simulink model "Areodynamic_Coefficient"  (R2022a)
settings: Solver=VariableStepAuto  StartTime=0.0  StopTime=1  RelTol=1e-3
undefined symbols (not defined in the file): a1, ac, AeroCoeff, b1
libraries: aerolibconvert2 x4
(part 2 of 2)

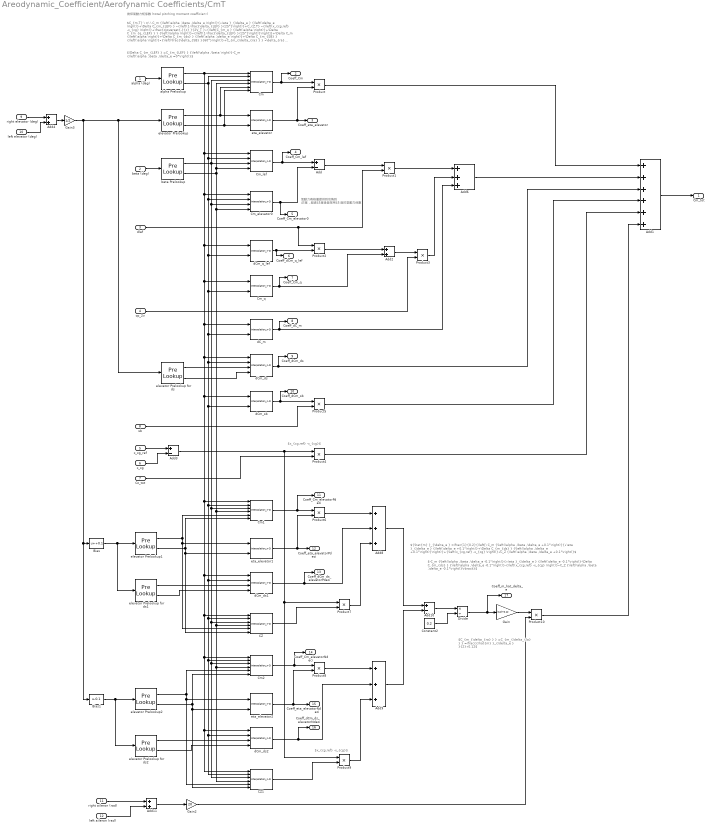
== system Areodynamic_Coefficient/Aerofynamic Coefficients/CmT ==
  note: 氣動力表格僅提供到攻角到
      | 45度，超過45度後皆採用45
      | 度的氣動力係數
  note: $x_{cg,ref} -x_{cg}$
  note: 俯仰氣動力矩係數 (total pitching moment coefficient)：
  note: $\Delta C_{m_{LEF} } =C_{m_{LEF} } {\left(\alpha ,\beta \right)}-C_m {\left(\alpha ,\beta ,\delta_e =0°\right)}$
  note: $C_{m,T} \ =\ \ C_m {\left(\alpha ,\beta ,\delta_e \right)}{∙\eta }_{\delta_e } {\left(\delta_e \right)}+\Delta C_{m_{LEF} } ∙{\left(1-\frac{\delta_{LEF} }{25°}\right)}+C_{Z,T} ∙{\left(x_{cg,ref} -x_{cg} \right)}+\frac{q\overset{-}{c} }{2V_T }∙{\left[C_{m_q } {\left(\alpha \right)}+\Delta C_{m_{q_{LEF} } } {\left(\alpha \right)}∙{\left(1-\frac{\delta_{LEF} }{25°}\right)}\right]}+\Delta C_m {\left(\alpha \right)}+\Delta C_{m_{ds} } {\left(\alpha ,\delta_e \right)}+\Delta C_{m_{SB} } {\left(\alpha \right)}∙{\left(\frac{\delta_{SB} }{60°}\right)}+C_{m_{\delta_{ra} } } ∙\delta_{ra} +C_{m_{\delta_{la} } } ∙\delta_{la}$
  note: $-C_m {\left(\alpha ,\beta ,\delta_e -0.1°\right)}{∙\eta }_{\delta_e } {\left(\delta_e -0.1°\right)}-\Delta C_{m_{ds} } {\left(\alpha ,\delta_e -0.1°\right)}-{\left(x_{cg,ref} -x_{cg} \right)}∙C_Z {\left(\alpha ,\beta ,\delta_e -0.1°\right)}\rbrack}$
  note: ${\hat{m} }_{\delta_e } =\frac{1}{0.2}{\left[\ C_m {\left(\alpha ,\beta ,\delta_e +0.1°\right)}{∙\eta }_{\delta_e } {\left(\delta_e +0.1°\right)}+\Delta C_{m_{ds} } {\left(\alpha ,\delta_e +0.1°\right)}\right)}+{\left(x_{cg,ref} -x_{cg} \right)}∙C_Z {\left(\alpha ,\beta ,\delta_e +0.1°\right)}$
  note: $x_{cg,ref} -x_{cg}$
  note: $C_{m_{\delta_{ra} } } =C_{m_{\delta_{la} } } =\frac{{\hat{m} }_{\delta_e } }{2}∙0.12$
  alpha (deg) : Inport
  beta (deg) : Inport  Port=2
  dlef : Inport  Port=3
  qc_2v : Inport  Port=4
  x_cg_ref : Inport  Port=5
  x_cg : Inport  Port=6
  Cz_tot : Inport  Port=7
  sb : Inport  Port=8
  right elevator (deg) : Inport  Port=9
  left elevator (deg) : Inport  Port=10
  right aileron (rad) : Inport  Port=11
  left aileron (rad) : Inport  Port=12
  Add : Sum  Inputs=+-
  Add1 : Sum  Inputs=++++++
  Add10 : Sum  Inputs=+-
  Add11 : Sum
  Add2 : Sum
  Add3 : Sum  Inputs=+-
  Add4 : Sum
  Add6 : Sum  Inputs=+++
  Add8 : Sum  Inputs=+++
  Add9 : Sum  Inputs=+++
  Bias : Bias  Bias=+0.1  SaturateOnIntegerOverflow=off
  Bias1 : Bias  Bias=-0.1  SaturateOnIntegerOverflow=off
  CZ : Interpolation_n-D  NumberOfTableDimensions=3  Table=AeroCoeff.CZ
      settings: InputPortMap=u0,u1,u2,u3,u4,u5
  CZ1 : Interpolation_n-D  NumberOfTableDimensions=3  Table=AeroCoeff.CZ
      settings: InputPortMap=u0,u1,u2,u3,u4,u5
  Cm : Interpolation_n-D  NumberOfTableDimensions=3  Table=AeroCoeff.Cm
      settings: InputPortMap=u0,u1,u2,u3,u4,u5
  Cm1 : Interpolation_n-D  NumberOfTableDimensions=3  Table=AeroCoeff.Cm
      settings: InputPortMap=u0,u1,u2,u3,u4,u5
  Cm2 : Interpolation_n-D  NumberOfTableDimensions=3  Table=AeroCoeff.Cm
      settings: InputPortMap=u0,u1,u2,u3,u4,u5
  Cm_elevator0 : Interpolation_n-D  Table=AeroCoeff.Cm_elevator0
  Cm_lef : Interpolation_n-D  Table=AeroCoeff.Cm_lef
  Cm_q : Interpolation_n-D  NumberOfTableDimensions=1  Table=AeroCoeff.Cm_q
      settings: InputPortMap=u0,u1
  Constant2 : Constant  Value=0.2
  Divide : Product  Inputs=*/
  Gain : Gain  Gain=(1/2)*0.12
  Gain2 : Gain  Gain=20
  Gain3 : Gain  Gain=1/2
  Product{,1..10} (11 alike) : Product
  alpha Prelookup : PreLookup  BreakpointsData=AeroCoeff.alpha_prelookup  IndexSearchMethod=Linear search  BeginIndexSearchUsingPreviousIndexResult=on  DiagnosticForOutOfRangeInput=Warning
  beta Prelookup : PreLookup  BreakpointsData=AeroCoeff.beta_prelookup  IndexSearchMethod=Linear search  BeginIndexSearchUsingPreviousIndexResult=on  DiagnosticForOutOfRangeInput=Warning
  dC_m : Interpolation_n-D  NumberOfTableDimensions=1  Table=AeroCoeff.dC_m
      settings: InputPortMap=u0,u1
  dCm_ds : Interpolation_n-D  Table=AeroCoeff.dCm_ds
  dCm_ds1 : Interpolation_n-D  Table=AeroCoeff.dCm_ds
  dCm_ds2 : Interpolation_n-D  Table=AeroCoeff.dCm_ds
  dCm_q_lef : Interpolation_n-D  NumberOfTableDimensions=1  Table=AeroCoeff.dCm_q_lef
      settings: InputPortMap=u0,u1
  dCm_sb : Interpolation_n-D  NumberOfTableDimensions=1  Table=AeroCoeff.dCm_sb
      settings: InputPortMap=u0,u1
  elevator Prelookup : PreLookup  BreakpointsData=AeroCoeff.elevator_prelookup2  IndexSearchMethod=Linear search  BeginIndexSearchUsingPreviousIndexResult=on  DiagnosticForOutOfRangeInput=Warning
  elevator Prelookup for ds : PreLookup  BreakpointsData=AeroCoeff.elevator_prelookup3  IndexSearchMethod=Linear search  BeginIndexSearchUsingPreviousIndexResult=on  DiagnosticForOutOfRangeInput=Warning
  elevator Prelookup for ds1 : PreLookup  BreakpointsData=AeroCoeff.elevator_prelookup3  IndexSearchMethod=Linear search  BeginIndexSearchUsingPreviousIndexResult=on  DiagnosticForOutOfRangeInput=Warning
  elevator Prelookup for ds2 : PreLookup  BreakpointsData=AeroCoeff.elevator_prelookup3  IndexSearchMethod=Linear search  BeginIndexSearchUsingPreviousIndexResult=on  DiagnosticForOutOfRangeInput=Warning
  elevator Prelookup1 : PreLookup  BreakpointsData=AeroCoeff.elevator_prelookup2  IndexSearchMethod=Linear search  BeginIndexSearchUsingPreviousIndexResult=on  DiagnosticForOutOfRangeInput=Warning
  elevator Prelookup2 : PreLookup  BreakpointsData=AeroCoeff.elevator_prelookup2  IndexSearchMethod=Linear search  BeginIndexSearchUsingPreviousIndexResult=on  DiagnosticForOutOfRangeInput=Warning
  eta_elevator : Interpolation_n-D  NumberOfTableDimensions=1  Table=AeroCoeff.eta_elevator
      settings: InputPortMap=u0,u1
  eta_elevator1 : Interpolation_n-D  NumberOfTableDimensions=1  Table=AeroCoeff.eta_elevator
      settings: InputPortMap=u0,u1
  eta_elevator2 : Interpolation_n-D  NumberOfTableDimensions=1  Table=AeroCoeff.eta_elevator
      settings: InputPortMap=u0,u1
  Cm_tot : Outport  VectorParamsAs1DForOutWhenUnconnected=off
  Coeff_Cm : Outport  Port=2
  Coeff_eta_elevator : Outport  Port=3
  Coeff_Cm_lef : Outport  Port=4
  Coeff_Cm_elevator0 : Outport  Port=5
  Coeff_dCm_q_lef : Outport  Port=6
  Coeff_Cm_q : Outport  Port=7
  Coeff_dC_m : Outport  Port=8
  Coeff_dCm_ds : Outport  Port=9
  Coeff_dCm_sb : Outport  Port=10
  Coeff_Cm_elevatorPdeci : Outport  Port=11
  Coeff_eta_elevatorPdeci : Outport  Port=12
  Coeff_dCm_ds_elevatorPdeci : Outport  Port=13
  Coeff_Cm_elevatorNdeci : Outport  Port=14
  Coeff_eta_elevatorNdeci : Outport  Port=15
  Coeff_dCm_ds_elevatorNdeci : Outport  Port=16
  Coeff_m_hat_delta_e : Outport  Port=17
  wires:
  Cm_lef/1 -> Coeff_Cm_lef/1, Add/1
  Add3/1 -> Product4/1, Product7/1, Product9/1
  alpha Prelookup/1 -> Cm1/1, dCm_ds2/1, CZ1/1, Cm2/1, CZ/1, dCm_ds1/1, dCm_sb/1, dCm_ds/1, dC_m/1, Cm_q/1, dCm_q_lef/1, Cm_elevator0/1, Cm_lef/1, Cm/1
  Cm_elevator0/1 -> Coeff_Cm_elevator0/1, Add/2
  elevator Prelookup/1 -> eta_elevator/1, Cm/5
  dC_m/1 -> Coeff_dC_m/1, Add6/3
  alpha Prelookup/2 -> Cm1/2, dCm_ds1/2, Cm2/2, dCm_ds2/2, CZ1/2, CZ/2, dCm_sb/2, dCm_ds/2, dC_m/2, Cm_q/2, dCm_q_lef/2, Cm_elevator0/2, Cm_lef/2, Cm/2
  dlef/1 -> Product2/1, Product1/2
  elevator Prelookup/2 -> eta_elevator/2, Cm/6
  Add4/1 -> Gain3/1
  eta_elevator/1 -> Coeff_eta_elevator/1, Product/2
  beta Prelookup/2 -> Cm/4, Cm_lef/4, Cm1/4, CZ/4, Cm2/4, CZ1/4, Cm_elevator0/4
  Product2/1 -> Add2/1
  Cm_q/1 -> Coeff_Cm_q/1, Add2/2
  beta Prelookup/1 -> Cm/3, Cm1/3, CZ/3, Cm2/3, CZ1/3, Cm_elevator0/3, Cm_lef/3
  dCm_q_lef/1 -> Coeff_dCm_q_lef/1, Product2/2
  Add2/1 -> Product3/1
  Add/1 -> Product1/1
  qc_2v/1 -> Product3/2
  alpha (deg)/1 -> alpha Prelookup/1
  Product4/1 -> Add1/5
  beta (deg)/1 -> beta Prelookup/1
  x_cg/1 -> Add3/2
  Add1/1 -> Cm_tot/1
  Cz_tot/1 -> Product4/2
  x_cg_ref/1 -> Add3/1
  sb/1 -> Product5/2
  dCm_sb/1 -> Coeff_dCm_sb/1, Product5/1
  Product5/1 -> Add1/4
  elevator Prelookup for ds/1 -> dCm_ds/3
  elevator Prelookup for ds/2 -> dCm_ds/4
  dCm_ds/1 -> Coeff_dCm_ds/1, Add1/3
  Product1/1 -> Add6/1
  Product3/1 -> Add6/2
  Add6/1 -> Add1/2
  Product/1 -> Add1/1
  right elevator (deg)/1 -> Add4/1
  left elevator (deg)/1 -> Add4/2
  eta_elevator1/1 -> Product6/2, Coeff_eta_elevatorPdeci/1
  Cm1/1 -> Coeff_Cm_elevatorPdeci/1, Product6/1
  elevator Prelookup1/1 -> Cm1/5, eta_elevator1/1, CZ/5
  elevator Prelookup1/2 -> Cm1/6, eta_elevator1/2, CZ/6
  Bias/1 -> elevator Prelookup1/1, elevator Prelookup for ds1/1
  elevator Prelookup for ds1/1 -> dCm_ds1/3
  elevator Prelookup for ds1/2 -> dCm_ds1/4
  Product6/1 -> Add8/1
  dCm_ds1/1 -> Coeff_dCm_ds_elevatorPdeci/1, Add8/2
  Product7/1 -> Add8/3
  Bias1/1 -> elevator Prelookup2/1, elevator Prelookup for ds2/1
  elevator Prelookup2/1 -> eta_elevator2/1, CZ1/5, Cm2/5
  elevator Prelookup2/2 -> eta_elevator2/2, CZ1/6, Cm2/6
  elevator Prelookup for ds2/1 -> dCm_ds2/3
  elevator Prelookup for ds2/2 -> dCm_ds2/4
  Cm2/1 -> Coeff_Cm_elevatorNdeci/1, Product8/1
  eta_elevator2/1 -> Coeff_eta_elevatorNdeci/1, Product8/2
  Product8/1 -> Add9/1
  dCm_ds2/1 -> Coeff_dCm_ds_elevatorNdeci/1, Add9/2
  CZ1/1 -> Product9/2
  Product9/1 -> Add9/3
  Add8/1 -> Add10/1
  Add9/1 -> Add10/2
  Add10/1 -> Divide/1
  Constant2/1 -> Divide/2
  Divide/1 -> Coeff_m_hat_delta_e/1, Gain/1
  Gain/1 -> Product10/1
  right aileron (rad)/1 -> Add11/1
  left aileron (rad)/1 -> Add11/2
  Add11/1 -> Gain2/1
  Product10/1 -> Add1/6
  Gain2/1 -> Product10/2
  Gain3/1 -> elevator Prelookup/1, elevator Prelookup for ds/1, Bias1/1, Bias/1
  Cm/1 -> Coeff_Cm/1, Product/1
  CZ/1 -> Product7/2

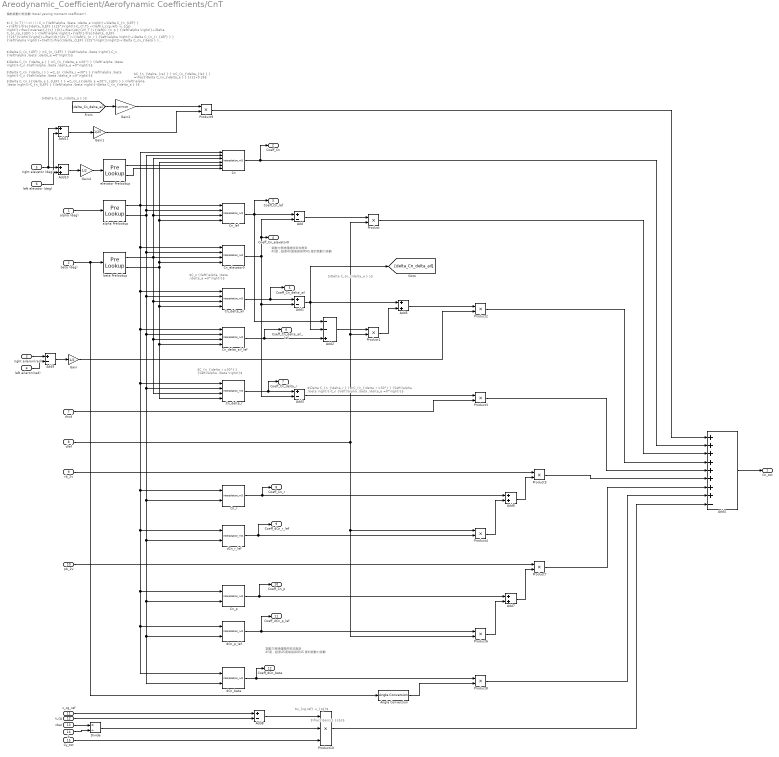
== system Areodynamic_Coefficient/Aerofynamic Coefficients/CnT ==
  note: $\Delta C_{n_{\delta_a } }$
  note: 氣動力表格僅提供到攻角到
      | 45度，超過45度後皆採用45
      | 度的氣動力係數
  note: 氣動力表格僅提供到攻角到
      | 45度，超過45度後皆採用45
      | 度的氣動力係數
  note: $C_n {\left(\alpha ,\beta ,\delta_e =0°\right)}$
  note: $C_{n_{\delta_r =30°} } {\left(\alpha ,\beta \right)}$
  note: $\Delta C_{n_{\delta_r } } =C_{n_{\delta_r =30°} } {\left(\alpha ,\beta \right)}-C_n {\left(\alpha ,\beta ,\delta_e =0°\right)}$
  note: $x_{cg,ref} -x_{cg}$
  note: $\frac{\bar{c} }{b}$
  note: $\Delta C_{n_{\delta_a } } =C_{n_{\delta_a =20°} } {\left(\alpha ,\beta \right)}-C_n {\left(\alpha ,\beta ,\delta_e =0°\right)}$
  note: $\Delta C_{n_{\delta_r } } =C_{n_{\delta_r =30°} } {\left(\alpha ,\beta \right)}-C_n {\left(\alpha ,\beta ,\delta_e =0°\right)}$
  note: $\ C_{n,T} \ \ =\ \ \ \ C_n {\left(\alpha ,\beta ,\delta_e \right)}+\Delta C_{n_{LEF} } ∙{\left(1-\frac{\delta_{LEF} }{25°}\right)}-C_{Y,T} ∙{\left(x_{cg,ref} -x_{cg} \right)}∙\frac{\overset{-}{c} }{b}+\frac{pb}{2V_T }∙{\left[C_{n_p } {\left(\alpha \right)}+\Delta C_{n_{p_{LEF} } } {\left(\alpha \right)}∙{\left(1-\frac{\delta_{LEF} }{25°}\right)}\right]}+\frac{rb}{2V_T }∙{\left[C_{n_r } {\left(\alpha \right)}+\Delta C_{n_{r_{LEF} } } {\left(\alpha \right)}∙{\left(1-\frac{\delta_{LEF} }{25°}\right)}\right]}+\Delta C_{n_{\beta } } {\left(\alpha \right)}∙\beta +\Delta C_{n_{\delta_r } } ∙{\left(\frac{\delta_r }{30°}\right)}+\frac{{\left[\Delta C_{n_{\delta_a } } +\Delta C_{n_{{\delta_a }_{LEF} } } ∙{\left(1-\frac{\delta_{LEF} }{25°}\right)}\right]}}{2}∙{\left(\frac{\delta_{ra} }{20°}\right)}-\frac{{\left[\Delta C_{n_{\delta_a } } +\Delta C_{n_{{\delta_a }_{LEF} } } ∙{\left(1-\frac{\delta_{LEF} }{25°}\right)}\right]}}{2}∙{\left(\frac{\delta_{la} }{20°}\right)}+C_{n_{\delta_{re} } } ∙{\left(\frac{\delta_{re} }{30°}\right)}-C_{n_{\delta_{le} } } ∙{\left(\frac{\delta_{le} }{30°}\right)}$
  note: $\Delta C_{n_{LEF} } =C_{n_{LEF} } {\left(\alpha ,\beta \right)}-C_n {\left(\alpha ,\beta ,\delta_e =0°\right)}$
  note: 偏航氣動力矩係數 (total yawing moment coefficient)：
  note: $\Delta C_{n_{{\delta_a }_{LEF} } } =C_{n_{{\delta_a =20°}_{LEF} } } {\left(\alpha ,\beta \right)}-C_{n_{LEF} } {\left(\alpha ,\beta \right)}-\Delta C_{n_{\delta_a } }$
  note: $\Delta C_{n_{\delta_a } }$
  note: $C_{n_{\delta_{re} } } =C_{n_{\delta_{le} } } =\frac{\Delta C_{n_{\delta_a } } }{2}∙0.26$
  alpha (deg) : Inport
  beta (deg) : Inport  Port=2
  right aileron(rad) : Inport  Port=3
  left aileron(rad) : Inport  Port=4
  "right elevator (deg) " : Inport  Port=5
  left elevator (deg) : Inport  Port=6
  drud : Inport  Port=7
  dlef : Inport  Port=8
  rb_2v : Inport  Port=9
  pb_2v : Inport  Port=10
  x_cg_ref : Inport  Port=11
  x_cg : Inport  Port=12
  cbar : Inport  Port=13
  b : Inport  Port=14
  Cy_tot : Inport  Port=15
  Add{,1,3,8..9,11} (6 alike) : Sum  Inputs=+-
  Add{5..7,10} (4 alike) : Sum
  Add2 : Sum  Inputs=--+
  Add4 : Sum  Inputs=++++++++-
  Angle Conversion : aerolibconvert2/Angle Conversion  IU=deg  OU=rad
  Cn : Interpolation_n-D  NumberOfTableDimensions=3  Table=AeroCoeff.Cn
      settings: InputPortMap=u0,u1,u2,u3,u4,u5
  Cn_delta_ail : Interpolation_n-D  Table=AeroCoeff.Cn_delta_ail
  Cn_delta_ail_lef : Interpolation_n-D  Table=AeroCoeff.Cn_delta_ail_lef
  Cn_delta_r : Interpolation_n-D  Table=AeroCoeff.Cn_delta_r
  Cn_elevator0 : Interpolation_n-D  Table=AeroCoeff.Cn_elevator0
  Cn_lef : Interpolation_n-D  Table=AeroCoeff.Cn_lef
  Cn_p : Interpolation_n-D  NumberOfTableDimensions=1  Table=AeroCoeff.Cn_p
      settings: InputPortMap=u0,u1
  Cn_r : Interpolation_n-D  NumberOfTableDimensions=1  Table=AeroCoeff.Cn_r
      settings: InputPortMap=u0,u1
  Divide : Product  Inputs=*/
  Gain : Gain  Gain=1/2
  Gain1 : Gain  Gain=1/25
  Gain2 : Gain  Gain=(1/2)*0.26
  Gain4 : Gain  Gain=1/2
  Product{,1..9} (10 alike) : Product
  Product10 : Product  Inputs=3
  alpha Prelookup : PreLookup  BreakpointsData=AeroCoeff.alpha_prelookup  IndexSearchMethod=Linear search  BeginIndexSearchUsingPreviousIndexResult=on  DiagnosticForOutOfRangeInput=Warning
  beta Prelookup : PreLookup  BreakpointsData=AeroCoeff.beta_prelookup  IndexSearchMethod=Linear search  BeginIndexSearchUsingPreviousIndexResult=on  DiagnosticForOutOfRangeInput=Warning
  dCn_beta : Interpolation_n-D  NumberOfTableDimensions=1  Table=AeroCoeff.dCn_beta
      settings: InputPortMap=u0,u1
  dCn_p_lef : Interpolation_n-D  NumberOfTableDimensions=1  Table=AeroCoeff.dCn_p_lef
      settings: InputPortMap=u0,u1
  dCn_r_lef : Interpolation_n-D  NumberOfTableDimensions=1  Table=AeroCoeff.dCn_r_lef
      settings: InputPortMap=u0,u1
  elevator Prelookup : PreLookup  BreakpointsData=AeroCoeff.elevator_prelookup1  IndexSearchMethod=Linear search  BeginIndexSearchUsingPreviousIndexResult=on  DiagnosticForOutOfRangeInput=Warning
  Cn_tot : Outport  VectorParamsAs1DForOutWhenUnconnected=off
  Coeff_Cn : Outport  Port=2
  Coeff_Cn_lef : Outport  Port=3
  Coeff_Cn_elevator0 : Outport  Port=4
  Coeff_Cn_delta_ail : Outport  Port=5
  Coeff_Cn_delta_ail_lef : Outport  Port=6
  Coeff_Cn_delta_r : Outport  Port=7
  Coeff_Cn_r : Outport  Port=8
  Coeff_dCn_r_lef : Outport  Port=9
  Coeff_Cn_p : Outport  Port=10
  Coeff_dCn_p_lef : Outport  Port=11
  Coeff_dCn_beta : Outport  Port=12
  wires:
  alpha Prelookup/1 -> Cn/1, dCn_p_lef/1, dCn_beta/1, Cn_p/1, dCn_r_lef/1, Cn_r/1, Cn_delta_r/1, Cn_delta_ail_lef/1, Cn_delta_ail/1, Cn_elevator0/1, Cn_lef/1
  Add1/1 -> Add5/1, [delta_Cn_delta_ail], Add2/2
  Cn_elevator0/1 -> Add3/2, Add1/2, Coeff_Cn_elevator0/1, Add/2
  alpha Prelookup/2 -> Cn/2, Cn_lef/2, dCn_p_lef/2, dCn_beta/2, Cn_p/2, dCn_r_lef/2, Cn_r/2, Cn_delta_r/2, Cn_delta_ail_lef/2, Cn_delta_ail/2, Cn_elevator0/2
  elevator Prelookup/1 -> Cn/5
  Add6/1 -> Product5/2
  beta Prelookup/2 -> Cn_delta_r/4, Cn_delta_ail_lef/4, Cn_delta_ail/4, Cn/4, Cn_lef/4, Cn_elevator0/4
  Cn_r/1 -> Coeff_Cn_r/1, Add6/1
  Cn_delta_ail_lef/1 -> Coeff_Cn_delta_ail_lef/1, Add2/3
  pb_2v/1 -> Product7/1
  Add5/1 -> Product2/1
  Cn_lef/1 -> Add/1, Coeff_Cn_lef/1, Add2/1
  Add4/1 -> Cn_tot/1
  Add7/1 -> Product7/2
  beta (deg)/1 -> beta Prelookup/1, Angle Conversion/1
  rb_2v/1 -> Product5/1
  Product10/1 -> Add4/9
  Add/1 -> Product/1
  x_cg/1 -> Add8/2
  alpha (deg)/1 -> alpha Prelookup/1
  b/1 -> Divide/2
  dCn_r_lef/1 -> Coeff_dCn_r_lef/1, Product4/2
  drud/1 -> Product3/2
  dCn_beta/1 -> Coeff_dCn_beta/1, Product8/1
  Product4/1 -> Add6/2
  Divide/1 -> Product10/2
  Product3/1 -> Add4/5
  x_cg_ref/1 -> Add8/1
  Cn_p/1 -> Coeff_Cn_p/1, Add7/1
  dCn_p_lef/1 -> Coeff_dCn_p_lef/1, Product6/1
  Product8/1 -> Add4/8
  elevator Prelookup/2 -> Cn/6
  Cn_delta_r/1 -> Coeff_Cn_delta_r/1, Add3/1
  Product6/1 -> Add7/2
  Cy_tot/1 -> Product10/3
  Product7/1 -> Add4/7
  Product5/1 -> Add4/6
  Add2/1 -> Product1/1
  beta Prelookup/1 -> Cn_delta_r/3, Cn_delta_ail_lef/3, Cn_delta_ail/3, Cn/3, Cn_lef/3, Cn_elevator0/3
  Product2/1 -> Add4/4
  Cn/1 -> Coeff_Cn/1, Add4/2
  Cn_delta_ail/1 -> Coeff_Cn_delta_ail/1, Add1/1
  Add3/1 -> Product3/1
  dlef/1 -> Product6/2, Product4/1, Product/2, Product1/2
  Product/1 -> Add4/3
  Product1/1 -> Add5/2
  cbar/1 -> Divide/1
  Add8/1 -> Product10/1
  right aileron(rad)/1 -> Add9/1
  left aileron(rad)/1 -> Add9/2
  Add9/1 -> Gain/1
  Gain/1 -> Product2/2
  Add10/1 -> Gain4/1
  [delta_Cn_delta_ail] -> Gain2/1
  Gain1/1 -> Product9/2
  Gain2/1 -> Product9/1
  Product9/1 -> Add4/1
  "right elevator (deg) "/1 -> Add11/1, Add10/1
  left elevator (deg)/1 -> Add11/2, Add10/2
  Add11/1 -> Gain1/1
  Gain4/1 -> elevator Prelookup/1
  Angle Conversion/1 -> Product8/2

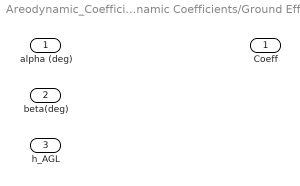
== system Areodynamic_Coefficient/Aerofynamic Coefficients/Ground Effects ==
  alpha (deg) : Inport
  beta(deg) : Inport  Port=2
  h_AGL : Inport  Port=3
  Coeff : Outport

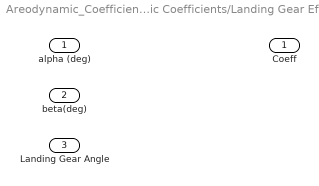
== system Areodynamic_Coefficient/Aerofynamic Coefficients/Landing Gear Effects ==
  alpha (deg) : Inport
  beta(deg) : Inport  Port=2
  Landing Gear Angle : Inport  Port=3
  Coeff : Outport
